simulink model "DC_DC_G13_sim_L1"  (R2024b)
settings: Solver=ode23tb  StartTime=0.0  StopTime=0.04  MaxStep=1/fpwm/200  RelTol=1e-3
undefined symbols (not defined in the file): Cf, fpwm, Lf, ri, Rmax, U
libraries: spsSeriesRLCBranchLib x5, spsCurrentMeasurementLib x3, spsMeanLib x3, spsVoltageMeasurementLib x3, spsBreakerLib x1, spsDiodeLib x1, spsMosfetLib x1, spsDCVoltageSourceLib x1, sps_lib x1
settings Model: Creator=Martinha  LastModifiedBy=franc

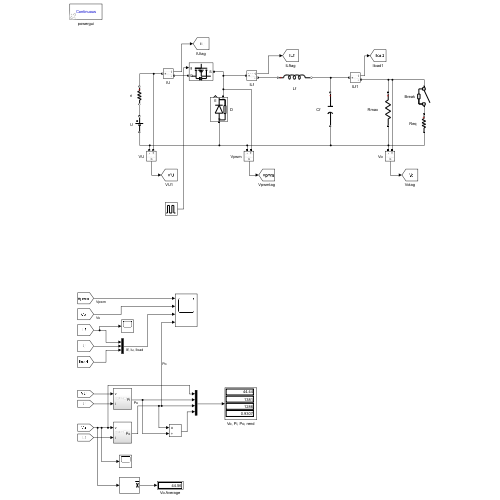
[thumbnail: Simulink's stored preview of the top-level diagram]
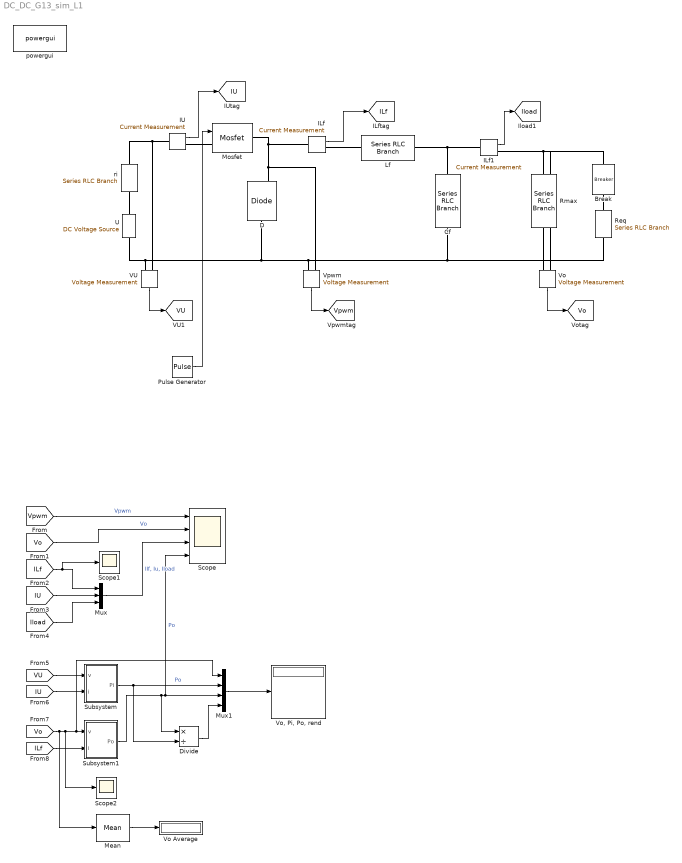
== system DC_DC_G13_sim_L1 ==
  Break : spsBreakerLib/Breaker  InitialState=0  SwitchingTimes=[0.02]  External=off  BreakerResistance=0.01  SnubberResistance=Rs  SnubberCapacitance=Cs  Measurements=None  MoreParameters=on  NoBreakLoop=off
  Cf : spsSeriesRLCBranchLib/Series RLC Branch  LConnTagsString=__new0  RConnTagsString=__new0  BranchType=C  Resistance=1  Inductance=1e-3  SetiL0=off  InitialCurrent=0  Capacitance=Cf  Setx0=off  InitialVoltage=0  Measurements=None
  D : spsDiodeLib/Diode  Ron=Ron  Lon=0  Vf=0.8  IC=0  UseSnubber=0  Rs=Rs  Cs=Cs  Measurements=on
  Divide : Product  Inputs=*/
  ILf : spsCurrentMeasurementLib/Current Measurement  PhasorSimulation=off  OutputType=Complex  PSBequivalent=0
  ILf1 : spsCurrentMeasurementLib/Current Measurement  PhasorSimulation=off  OutputType=Complex  PSBequivalent=0
  IU : spsCurrentMeasurementLib/Current Measurement  PhasorSimulation=off  OutputType=Complex  PSBequivalent=0
  Lf : spsSeriesRLCBranchLib/Series RLC Branch  LConnTagsString=__new0  RConnTagsString=__new0  BranchType=L  Resistance=1  Inductance=Lf  SetiL0=off  InitialCurrent=0  Capacitance=1e-6  Setx0=off  InitialVoltage=0  Measurements=None
  Mean : spsMeanLib/Mean  Freq=fpwm/10  Vinit=110  Ts=0
  Mosfet : spsMosfetLib/Mosfet  Ron=0.1  Lon=0  Rd=0.01  Vfd=0  IC=0  Rs=1e5  Cs=inf  Measurements=off
  Mux : Mux  Inputs=3
  Mux1 : Mux
  Pulse Generator : DiscretePulseGenerator  PulseType=Time based  Period=1e-4  PulseWidth=48
  Req : spsSeriesRLCBranchLib/Series RLC Branch  LConnTagsString=__new0  RConnTagsString=__new0  BranchType=R  Resistance=Rmax/14  Inductance=1e-3  SetiL0=off  InitialCurrent=0  Capacitance=1e-6  Setx0=off  InitialVoltage=0  Measurements=None
  Rmax : spsSeriesRLCBranchLib/Series RLC Branch  LConnTagsString=__new0  RConnTagsString=__new0  BranchType=R  Resistance=Rmax  Inductance=1e-3  SetiL0=off  InitialCurrent=0  Capacitance=1e-6  Setx0=off  InitialVoltage=0  Measurements=None
  Scope : Scope  NumInputPorts=4
  Scope1 : Scope
  Scope2 : Scope
  Subsystem : Subsystem
  Subsystem1 : Subsystem
  U : spsDCVoltageSourceLib/DC Voltage Source  Amplitude=U  Measurements=None
  VU : spsVoltageMeasurementLib/Voltage Measurement  PhasorSimulation=off  OutputType=Complex  PSBequivalent=0
  Vo : spsVoltageMeasurementLib/Voltage Measurement  PhasorSimulation=off  OutputType=Complex  PSBequivalent=0
  Vo Average : Display
  "Vo, Pi, Po, rend" : Display
  Vpwm : spsVoltageMeasurementLib/Voltage Measurement  PhasorSimulation=off  OutputType=Complex  PSBequivalent=0
  powergui : sps_lib/powergui  Priority=1  SimulationMode=Continuous  SampleTime=50e-6  frequency=60  Iterations=50  frequencyindice=0  Pbase=100e6  ErrMax=1e-4  UnitsV=kV  UnitsW=MW  buscounter=0  FunctionMessages=off  echomessages=off  EnableUseOfTLC=off  CurrentSourceSwitches=off  DisableSnubberDevices=off  DisableRonSwitches=off  DisableVfSwitches=off  DisplayEquations=off  AutomaticDiscreteSolvers=off  SolverType=Tustin/Backward Euler (TBE)  Interpol=off  ExternalGateDelay=off  methode=off  Ts=100  x0status=blocks  SPID=on  SwTol=0  HookPort=off  NonlinearTolerance=1e-4  nMaxIteration=100  ContinueOnMaxIteration=off  RestoreLinks=warning  ResistiveCurrentMeasurement=off  Frange=[0:2:500]  Ylog=off  Xlog=on  ShowGrid=off  save=off  variable=ZData  structure=0  ZoomFFT=off  StartTime=0.0  cycles=1  DisplayStyle=1  fundamental=60  FreqAxis=off  MaxFrequency=1000  frequencyindicesteady=1  RmsSteady=1  display=off
  ri : spsSeriesRLCBranchLib/Series RLC Branch  LConnTagsString=__new0  RConnTagsString=__new0  BranchType=R  Resistance=ri  Inductance=1e-3  SetiL0=off  InitialCurrent=0  Capacitance=1e-6  Setx0=off  InitialVoltage=0  Measurements=None
  tag scope: ILf=global, IU=global, Iload=global, VU=global, Vo=global, Vpwm=global
  wires:
  IU/1 -> [IU]
  VU/1 -> [VU]
  Vpwm/1 -> [Vpwm]
  Vo/1 -> [Vo]
  ILf1/1 -> [Iload]
  ILf/1 -> [ILf]
  Pulse Generator/1 -> Mosfet/1
  [ILf] -> Scope1/1, Mux/1
  [IU] -> Mux/2
  [Iload] -> Mux/3
  [VU] -> Subsystem/1(v)
  [IU] -> Subsystem/2(i)
  [ILf] -> Subsystem1/2(i)
  Subsystem/1(Pi) -> Divide/2, Mux1/2  "Po"
  Subsystem1/1(Po) -> Scope/4, Mux1/3, Divide/1  "Po"
  Mux1/1 -> "Vo, Pi, Po, rend"/1
  Divide/1 -> Mux1/4
  [Vpwm] -> Scope/1  "Vpwm"
  Mux/1 -> Scope/3  "Ilf, Iu, Iload"
  [Vo] -> Mean/1, Scope2/1, Mux1/1, Subsystem1/1(v)
  [Vo] -> Scope/2  "Vo"
  Mean/1 -> Vo Average/1
  connections:
  Lf/RConn1 -- ILf1/LConn1 -- Cf/LConn1
  Mosfet/RConn1 -- Vpwm/LConn1 -- D/RConn1 -- ILf/LConn1
  U/LConn1 -- VU/LConn2 -- Req/RConn1 -- Rmax/RConn1 -- Vo/LConn2 -- Cf/RConn1 -- Vpwm/LConn2 -- D/LConn1
  IU/RConn1 -- Mosfet/LConn1
  ri/RConn1 -- U/RConn1
  VU/LConn1 -- ri/LConn1 -- IU/LConn1
  ILf/RConn1 -- Lf/LConn1
  Rmax/LConn1 -- Break/LConn1 -- Vo/LConn1 -- ILf1/RConn1
  Req/LConn1 -- Break/RConn1

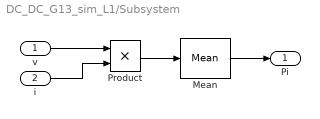
== system DC_DC_G13_sim_L1/Subsystem ==
  v : Inport
  i : Inport  Port=2
  Mean : spsMeanLib/Mean  Freq=fpwm/10  Vinit=110  Ts=0
  Product : Product
  Pi : Outport
  wires:
  Mean/1 -> Pi/1
  i/1 -> Product/2
  v/1 -> Product/1
  Product/1 -> Mean/1

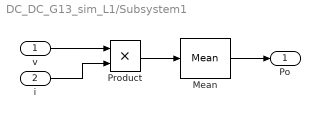
== system DC_DC_G13_sim_L1/Subsystem1 ==
  v : Inport
  i : Inport  Port=2
  Mean : spsMeanLib/Mean  Freq=fpwm/10  Vinit=110  Ts=0
  Product : Product
  Po : Outport
  wires:
  Mean/1 -> Po/1
  i/1 -> Product/2
  v/1 -> Product/1
  Product/1 -> Mean/1
